simulink model "hastighedsregulering"  (Simulink 7.4)
settings: Solver=ode45  StartTime=0.0  StopTime=10.0  RelTol=1e-3
values from neighbouring files (symbols this model uses):
  Bs = 1.748817703686052e-04    (= 0.000174881770369)    [armposregdimensionering.m]    (also in armposregsimuStart.m; hastighedsreguleringStart.m; hastregDimensionering.m; pindposregdimensionering.m)
  initU = 1.7    [armposregsimuStart.m]    (also in hastighedsreguleringStart.m; pindregStart.m)
  Js = 2.686970843428432e-04    (= 0.000268697084343)    [armposregdimensionering.m]    (also in armposregsimuStart.m; hastighedsreguleringStart.m; hastregDimensionering.m; pindposregdimensionering.m)
  Km = 0.022141706562986    (= 0.022141706563)    [armposregdimensionering.m]    (also in armposregsimuStart.m; hastighedsreguleringStart.m; hastregDimensionering.m; pindposregdimensionering.m)
  la = 0.3384    [armposregdimensionering.m]    (also in armposregsimuStart.m; hastighedsreguleringStart.m; hastregDimensionering.m; pindposregdimensionering.m)
  ma = 0.2988    [armposregdimensionering.m]    (also in armposregsimuStart.m = 0.298; hastighedsreguleringStart.m = 0.298; hastregDimensionering.m; pindposregdimensionering.m)
  N = 12/40    (= 0.3)    [armposregdimensionering.m]    (also in armposregsimuStart.m; hastighedsreguleringStart.m; hastregDimensionering.m; pindposregdimensionering.m)
  Rm = 0.807790757873553    (= 0.807790757874)    [armposregdimensionering.m]    (also in armposregsimuStart.m; hastighedsreguleringStart.m; hastregDimensionering.m; pindposregdimensionering.m)
  tauc = 0.064    [hastighedsreguleringStart.m]
settings Model: Creator=Skov  LastModifiedBy=HOSTRUP

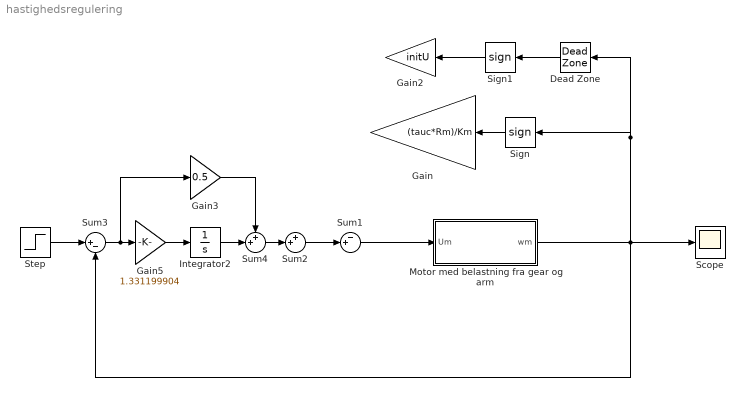
== system hastighedsregulering ==
  Dead Zone : DeadZone  LowerValue=-0.01  UpperValue=0.01  SampleTime=0.01  SaturateOnIntegerOverflow=on
  Gain : Gain  Gain=(tauc*Rm)/Km  ParameterDataType=fixdt(1, 16)  ParameterScaling=2^0  OutDataType=fixdt(1, 16)  OutScaling=2^0
  Gain2 : Gain  Gain=initU  ParameterDataType=fixdt(1, 16)  ParameterScaling=2^0  OutDataType=fixdt(1, 16)  OutScaling=2^0
  Gain3 : Gain  Gain=0.5  ParameterDataType=fixdt(1, 16)  ParameterScaling=2^0  OutDataType=fixdt(1, 16)  OutScaling=2^0
  Gain5 : Gain  Gain=1.331199904  ParameterDataType=fixdt(1, 16)  ParameterScaling=2^0  OutDataType=fixdt(1, 16)  OutScaling=2^0
  Integrator2 : Integrator
  Motor med belastning fra gear og arm : Subsystem
  Scope : Scope
  Sign : Signum  SampleTime=0.01
  Sign1 : Signum  SampleTime=0.01
  Step : Step  After=100  SampleTime=0
  Sum1 : Sum  Inputs=-+|  OutDataType=fixdt(1, 16)  OutScaling=2^0
  Sum2 : Sum  Inputs=++|  OutDataType=fixdt(1, 16)  OutScaling=2^0
  Sum3 : Sum  Inputs=|+-  OutDataType=fixdt(1, 16)  OutScaling=2^0
  Sum4 : Sum  Inputs=++|  OutDataType=fixdt(1, 16)  OutScaling=2^0
  wires:
  Motor med belastning fra gear og arm/1(wm) -> Scope/1, Sum3/2, Sign/1, Dead Zone/1
  Sum1/1 -> Motor med belastning fra gear og arm/1(Um)
  Sign/1 -> Gain/1
  Step/1 -> Sum3/1
  Sum2/1 -> Sum1/2
  Sign1/1 -> Gain2/1
  Gain5/1 -> Integrator2/1
  Integrator2/1 -> Sum4/2
  Gain3/1 -> Sum4/1
  Sum3/1 -> Gain5/1, Gain3/1
  Sum4/1 -> Sum2/2
  Dead Zone/1 -> Sign1/1

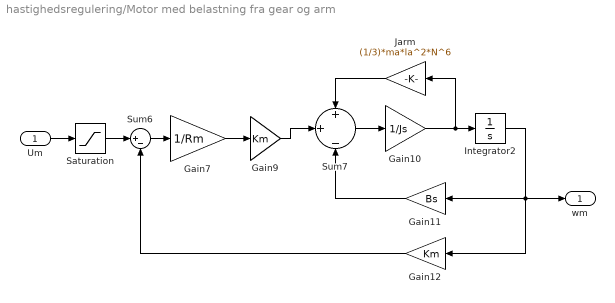
== system hastighedsregulering/Motor med belastning fra gear og arm ==
  Um : Inport  OutDataType=fixdt(1, 16)  OutScaling=2^0
  Gain10 : Gain  Gain=1/Js  ParameterDataType=fixdt(1, 16)  ParameterScaling=2^0  OutDataType=fixdt(1, 16)  OutScaling=2^0
  Gain11 : Gain  Gain=Bs  ParameterDataType=fixdt(1, 16)  ParameterScaling=2^0  OutDataType=fixdt(1, 16)  OutScaling=2^0
  Gain12 : Gain  Gain=Km  ParameterDataType=fixdt(1, 16)  ParameterScaling=2^0  OutDataType=fixdt(1, 16)  OutScaling=2^0
  Gain7 : Gain  Gain=1/Rm  ParameterDataType=fixdt(1, 16)  ParameterScaling=2^0  OutDataType=fixdt(1, 16)  OutScaling=2^0
  Gain9 : Gain  Gain=Km  ParameterDataType=fixdt(1, 16)  ParameterScaling=2^0  OutDataType=fixdt(1, 16)  OutScaling=2^0
  Integrator2 : Integrator
  Jarm : Gain  Gain=(1/3)*ma*la^2*N^6  ParameterDataType=fixdt(1, 16)  ParameterScaling=2^0  OutDataType=fixdt(1, 16)  OutScaling=2^0
  Saturation : Saturate  UpperLimit=13  LowerLimit=-13  OutDataType=fixdt(1, 16)  OutScaling=2^0
  Sum6 : Sum  Inputs=|+-  OutDataType=fixdt(1, 16)  OutScaling=2^0
  Sum7 : Sum  Inputs=+|+|-  OutDataType=fixdt(1, 16)  OutScaling=2^0
  wm : Outport  OutDataType=fixdt(1, 16)  OutScaling=2^0
  wires:
  Sum6/1 -> Gain7/1
  Gain7/1 -> Gain9/1
  Gain10/1 -> Integrator2/1, Jarm/1
  Sum7/1 -> Gain10/1
  Integrator2/1 -> Gain11/1, Gain12/1, wm/1
  Gain12/1 -> Sum6/2
  Saturation/1 -> Sum6/1
  Jarm/1 -> Sum7/1
  Um/1 -> Saturation/1
  Gain9/1 -> Sum7/2
  Gain11/1 -> Sum7/3
